simulink library "inp"  (R2021b)
settings: Solver=VariableStepAuto  StartTime=0.0  StopTime=10.0  RelTol=1e-3
undefined symbols (not defined in the file): C_TASK_5MS_S, FALSE, KINP_AcoreReadyToSlp_flg_ovrdflg, KINP_AcoreReadyToSlp_flg_ovrdval, KINP_AllowMovThd_OTA_enum_ovrdflg, KINP_AllowMovThd_OTA_enum_ovrdval, KINP_APSAngleTarget_Deg_ovrdflg, KINP_APSAngleTarget_Deg_ovrdval, KINP_APSDecReq_mps2_ovrdflg, KINP_APSDecReq_mps2_ovrdval, KINP_APSDecReqA_flg_ovrdflg, KINP_APSDecReqA_flg_ovrdval, KINP_APSDFLL_cm_ovrdflg, KINP_APSDFLL_cm_ovrdval, KINP_APSDFLR_cm_ovrdflg, KINP_APSDFLR_cm_ovrdval, KINP_APSDRLL_cm_ovrdflg, KINP_APSDRLL_cm_ovrdval, KINP_APSDRLR_cm_ovrdflg, KINP_APSDRLR_cm_ovrdval, KINP_APSExitCondition_enum_ovrdflg, KINP_APSExitCondition_enum_ovrdval, KINP_APSHWVer_enum_ovrdflg, KINP_APSHWVer_enum_ovrdval, KINP_APSProgressPCT_pct_ovrdflg, KINP_APSProgressPCT_pct_ovrdval, KINP_APSPwrReq_enum_ovrdflg, KINP_APSPwrReq_enum_ovrdval, KINP_APSReq_enum_ovrdflg, KINP_APSReq_enum_ovrdval, KINP_APSRQDisplay_enum_ovrdflg, KINP_APSRQDisplay_enum_ovrdval, KINP_APSRqEPASCtrl_flg_ovrdflg, KINP_APSRqEPASCtrl_flg_ovrdval, KINP_APSShiftPosnReq_enum_ovrdval, KINP_APSShiftPosnReq_enum_ovrflg, KINP_APSSpeedCMD_kph_ovrdval, KINP_APSSpeedCMD_kph_ovrflg, KINP_APSStaSystem_enum_ovrdflg, KINP_APSStaSystem_enum_ovrdval, KINP_APSSWVer_enum_ovrdflg, KINP_APSSWVer_enum_ovrdval, KINP_APSVMCReqA_flg_ovrdval, KINP_APSVMCReqA_flg_ovrflg, KINP_APSVRqEPASCtrl_flg_ovrdflg, KINP_APSVRqEPASCtrl_flg_ovrdval, KINP_AuxBattVolmV_mV_ovrdflg, KINP_AuxBattVolmV_mV_ovrdval, KINP_CAASSta_enum_ovrdflg, KINP_CAASSta_enum_ovrdval, KINP_CAASVMCReqA_flg_ovrdval, KINP_CAASVMCReqA_flg_ovrflg, KINP_CAN1BusOff_flg_ovrdflg, KINP_CAN1BusOff_flg_ovrdval, KINP_CAN2BusOff_flg_ovrdflg, KINP_CAN2BusOff_flg_ovrdval, KINP_CAN3BusOff_flg_ovrdflg, KINP_CAN3BusOff_flg_ovrdval, KINP_CAN4BusOff_flg_ovrdflg, KINP_CAN4BusOff_flg_ovrdval ... (+152)
libraries: FVT_lib x1037, hcu_lib x1
(part 1 of 34)
settings Model: Creator=13168  LastModifiedBy=FVT23118
settings SolverCC: AlgebraicLoopSolver=TrustRegion
settings DataIOCC: SaveFormat=Array  SignalLoggingSaveFormat=ModelDataLogs  ReturnWorkspaceOutputs=off
settings OptimizationCC: BlockReduction=off  BooleanDataType=off
settings DebuggingCC: SaveWithParameterizedLinksMsg=none  UnderspecifiedInitializationDetection=Classic  MergeDetectMultiDrivingBlocksExec=none  SignalResolutionControl=TryResolveAllWithWarning  SFMachineParentedDataDiag=warning
settings HardwareCC: TargetUnknown=on
settings ModelReferenceCC: PropagateSignalLabelsOutOfModel=off
settings SFSimCC: SimUseLocalCustomCode=off
settings ConfigComp: CovMetricSettings=dw  CovSaveCumulativeToWorkspaceVar=on  CovSaveSingleToWorkspaceVar=on

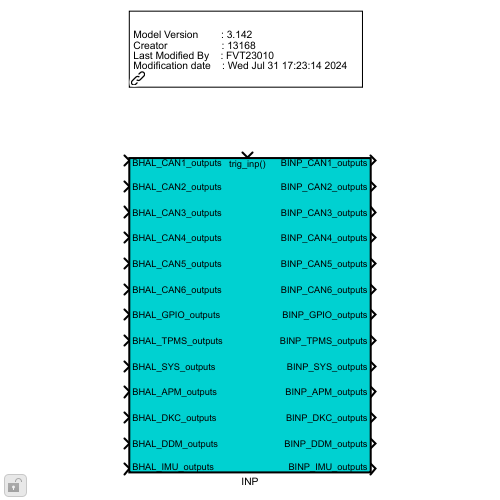
[thumbnail: Simulink's stored preview of the top-level diagram]
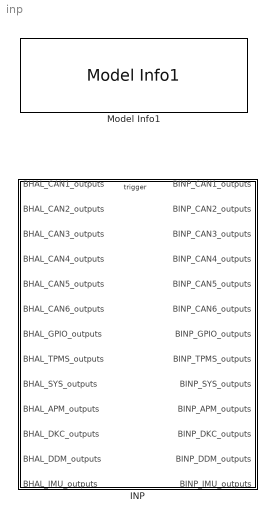
== system inp ==
  INP : Subsystem  TreatAsAtomicUnit=on
      settings: RTWSystemCode=Nonreusable function  RTWFcnNameOpts=Use subsystem name  RTWFileNameOpts=Use subsystem name
  Model Info1 : hcu_lib/Model Info1  BlockCM=None  Frame=on  DisplayStringWithTags=|  HorizontalTextAlignment=Left  LeftAlignmentValue=0.02  SourceBlockDiagram=hcu_lib  TagMaxNumber=20
      | Model Version        : %<ModelVersion>
      | Creator                   : %<Creator>
      | Last Modified By    : %<LastModifiedBy>
      | Modification date    : %<LastModificationDate>
      settings: SourceProductName=HCU Relative Block Library

== system inp/INP ==
  BHAL_CAN1_outputs : Inport  OutDataTypeStr=Bus: BHAL_CAN1_outputs
  BHAL_CAN2_outputs : Inport  Port=2  OutDataTypeStr=Bus: BHAL_CAN2_outputs
  BHAL_CAN3_outputs : Inport  Port=3  OutDataTypeStr=Bus: BHAL_CAN3_outputs
  BHAL_CAN4_outputs : Inport  Port=4  OutDataTypeStr=Bus: BHAL_CAN4_outputs
  BHAL_CAN5_outputs : Inport  Port=5  OutDataTypeStr=Bus: BHAL_CAN5_outputs
  BHAL_CAN6_outputs : Inport  Port=6  OutDataTypeStr=Bus: BHAL_CAN6_outputs
  BHAL_GPIO_outputs : Inport  Port=7  OutDataTypeStr=Bus: BHAL_GPIO_outputs
  BHAL_TPMS_outputs : Inport  Port=8  OutDataTypeStr=Bus: BHAL_TPMS_outputs
  BHAL_SYS_outputs : Inport  Port=9  OutDataTypeStr=Bus: BHAL_SYS_outputs
  BHAL_APM_outputs : Inport  Port=10  OutDataTypeStr=Bus: BHAL_APM_outputs
  BHAL_DKC_outputs : Inport  Port=11  OutDataTypeStr=Bus: BHAL_DKC_outputs
  BHAL_DDM_outputs : Inport  Port=12  OutDataTypeStr=Bus: BHAL_DDM_outputs
  BHAL_IMU_outputs : Inport  Port=13  OutDataTypeStr=Bus: BHAL_IMU_outputs
  trig_inp : TriggerPort  TriggerType=function-call  VariantControl=(inherit)
  APM : Subsystem
  CAN1 : Subsystem
  CAN2 : Subsystem
  CAN3 : Subsystem
  CAN4 : Subsystem
  CAN5 : Subsystem
  CAN6 : Subsystem
  DDM : Subsystem
  DKC : Subsystem
  GPIO : Subsystem
  IMU : Subsystem
  SYS : Subsystem
  TPMS : Subsystem
  BINP_CAN1_outputs : Outport  OutDataTypeStr=Bus: BINP_CAN1_outputs
  BINP_CAN2_outputs : Outport  Port=2  OutDataTypeStr=Bus: BINP_CAN2_outputs
  BINP_CAN3_outputs : Outport  Port=3  OutDataTypeStr=Bus: BINP_CAN3_outputs
  BINP_CAN4_outputs : Outport  Port=4  OutDataTypeStr=Bus: BINP_CAN4_outputs
  BINP_CAN5_outputs : Outport  Port=5  OutDataTypeStr=Bus: BINP_CAN5_outputs
  BINP_CAN6_outputs : Outport  Port=6  OutDataTypeStr=Bus: BINP_CAN6_outputs
  BINP_GPIO_outputs : Outport  Port=7  OutDataTypeStr=Bus: BINP_GPIO_outputs
  BINP_TPMS_outputs : Outport  Port=8  OutDataTypeStr=Bus: BINP_TPMS_outputs
  BINP_SYS_outputs : Outport  Port=9  OutDataTypeStr=Bus: BINP_SYS_outputs
  BINP_APM_outputs : Outport  Port=10  OutDataTypeStr=Bus: BINP_APM_outputs
  BINP_DKC_outputs : Outport  Port=11  OutDataTypeStr=Bus: BINP_DKC_outputs
  BINP_DDM_outputs : Outport  Port=12  OutDataTypeStr=Bus: BINP_DDM_outputs
  BINP_IMU_outputs : Outport  Port=13  OutDataTypeStr=Bus: BINP_IMU_outputs
  wires:
  BHAL_CAN1_outputs/1 -> CAN1/1(BHAL_CAN1_outputs)
  CAN1/1(INP_CAN1_outputs) -> BINP_CAN1_outputs/1
  BHAL_CAN2_outputs/1 -> CAN2/1(BHAL_CAN2_outputs)
  CAN2/1(INP_CAN2_outputs) -> BINP_CAN2_outputs/1
  BHAL_CAN3_outputs/1 -> CAN3/1(BHAL_CAN3_outputs)
  CAN3/1(INP_CAN3_outputs) -> BINP_CAN3_outputs/1
  BHAL_CAN4_outputs/1 -> CAN4/1(BHAL_CAN4_outputs)
  CAN4/1(INP_CAN4_outputs) -> BINP_CAN4_outputs/1
  GPIO/1(INP_GPIO_outputs) -> BINP_GPIO_outputs/1
  CAN5/1(INP_CAN5_outputs) -> BINP_CAN5_outputs/1
  BHAL_CAN5_outputs/1 -> CAN5/1(BHAL_CAN5_outputs)
  BHAL_GPIO_outputs/1 -> GPIO/1(BHAL_GPIO_outputs)
  BHAL_TPMS_outputs/1 -> TPMS/1(BHAL_TPMS_outputs)
  TPMS/1(BINP_TPMS_outputs) -> BINP_TPMS_outputs/1
  SYS/1(BINP_SYS_outputs) -> BINP_SYS_outputs/1
  BHAL_SYS_outputs/1 -> SYS/1(BHAL_SYS_outputs)
  BHAL_APM_outputs/1 -> APM/1(BHAL_APM_outputs)
  APM/1(BINP_APM_outputs) -> BINP_APM_outputs/1
  BHAL_DKC_outputs/1 -> DKC/1(BHAL_DKC_outputs)
  DKC/1(BINP_DKC_outputs) -> BINP_DKC_outputs/1
  BHAL_DDM_outputs/1 -> DDM/1(BHAL_DDM_outputs)
  DDM/1(BINP_DDM_outputs) -> BINP_DDM_outputs/1
  BHAL_IMU_outputs/1 -> IMU/1(BHAL_IMU_outputs)
  IMU/1(BINP_IMU_outputs) -> BINP_IMU_outputs/1
  BHAL_CAN6_outputs/1 -> CAN6/1(BHAL_CAN6_outputs)
  CAN6/1(INP_CAN6_outputs) -> BINP_CAN6_outputs/1

== system inp/INP/APM ==
  BHAL_APM_outputs : Inport  OutDataTypeStr=Bus: BHAL_APM_outputs
  Bus Creator : BusCreator  Inputs=58
  Bus Selector : BusSelector  OutputSignals=VHAL_PASDRMR_cm,VHAL_PASDRML_cm,VHAL_PASDRCR_cm,VHAL_PASDRCL_cm,VHAL_PASDFMR_cm,VHAL_PASDFML_cm,VHAL_PASDFCR_cm,VHAL_PASDFCL_cm,VHAL_APSDRLR_cm,VHAL_APSDRLL_cm,VHAL_APSDFLR_cm,VHAL_APSDFLL_cm,VHAL_PASAFCL_enum,VHAL_PASARMR_enum,VHAL_PASARML_enum,VHAL_PASARCR_enum,VHAL_PASARCL_enum,VHAL_PASAFMR_enum,VHAL_PASAFML_enum,VHAL_PASAFCR_enum,VHAL_USSStaRMR_flg,VHAL_USSStaRML_flg,VHAL_USSStaRLR_flg,VHAL_USSStaRLL_flg,VHAL_USSStaRCR_flg,VHAL_USSStaRCL_flg,VHAL_USSStaFMR_flg,VHAL_USSStaFML_flg,VHAL_USSStaFLR_flg,VHAL_USSStaFLL_flg,VHAL_USSStaFCR_flg,VHAL_USSStaFCL_flg,VHAL_Chime_enum,VHAL_SNSRLayout_enum,VHAL_StaFSya_flg,VHAL_ModOperation_enum,VHAL_APSProgressPCT_pct,VHAL_APSRQDisplay_enum,VHAL_APSSWVer_enum,VHAL_APSHWVer_enum,VHAL_APSExitCondition_enum,VHAL_APSAngleTarget_Deg,VHAL_APSStaSystem_enum,VHAL_APSVRqEPASCtrl_flg,VHAL_APSRqEPASCtrl_flg,VHAL_APSReq_enum,VHAL_APSDecReq_mps2,VHAL_APSDecReqA_flg,VHAL_APSShiftPosnReq_enum,VHAL_APSSpeedCMD_kph,VHAL_APSVMCReqA_flg,VHAL_CAASSta_enum,VHAL_CAASVMCReqA_flg,VHAL_APSPwrReq_enum,VHAL_RAPSBCMLockReq_flg,VHAL_RAPSBCMLamp_enum,VHAL_RAPSErrWarnSta_enum,VHAL_RAPSErrLv1_flg
  Data Type Conversion{,16,18..19,21..24,28..33,37,47..48,51,54,57} (20 alike) : DataTypeConversion  OutDataTypeStr=boolean
  Data Type Conversion{1..7,12..15,17,20,25..27,34..36,38,41..44,46,49,52..53,55..56} (30 alike) : DataTypeConversion  OutDataTypeStr=uint8
  Data Type Conversion{8..11} (4 alike) : DataTypeConversion  OutDataTypeStr=uint16
  Data Type Conversion{39..40,45,50} (4 alike) : DataTypeConversion  OutDataTypeStr=single
  Subsystem : Subsystem
  Subsystem1 : Subsystem
  Subsystem10 : Subsystem
  Subsystem11 : Subsystem
  Subsystem12 : Subsystem
  Subsystem13 : Subsystem
  Subsystem14 : Subsystem
  Subsystem15 : Subsystem
  Subsystem16 : Subsystem
  Subsystem17 : Subsystem
  Subsystem18 : Subsystem
  Subsystem19 : Subsystem
  Subsystem2 : Subsystem
  Subsystem20 : Subsystem
  Subsystem21 : Subsystem
  Subsystem22 : Subsystem
  Subsystem23 : Subsystem
  Subsystem24 : Subsystem
  Subsystem25 : Subsystem
  Subsystem26 : Subsystem
  Subsystem27 : Subsystem
  Subsystem28 : Subsystem
  Subsystem29 : Subsystem
  Subsystem3 : Subsystem
  Subsystem30 : Subsystem
  Subsystem31 : Subsystem
  Subsystem32 : Subsystem
  Subsystem33 : Subsystem
  Subsystem34 : Subsystem
  Subsystem35 : Subsystem
  Subsystem36 : Subsystem
  Subsystem37 : Subsystem
  Subsystem38 : Subsystem
  Subsystem39 : Subsystem
  Subsystem4 : Subsystem
  Subsystem40 : Subsystem
  Subsystem41 : Subsystem
  Subsystem42 : Subsystem
  Subsystem43 : Subsystem
  Subsystem44 : Subsystem
  Subsystem45 : Subsystem
  Subsystem46 : Subsystem
  Subsystem47 : Subsystem
  Subsystem48 : Subsystem
  Subsystem49 : Subsystem
  Subsystem5 : Subsystem
  Subsystem50 : Subsystem
  Subsystem51 : Subsystem
  Subsystem52 : Subsystem
  Subsystem53 : Subsystem
  Subsystem54 : Subsystem
  Subsystem55 : Subsystem
  Subsystem56 : Subsystem
  Subsystem57 : Subsystem
  Subsystem6 : Subsystem
  Subsystem7 : Subsystem
  Subsystem8 : Subsystem
  Subsystem9 : Subsystem
  BINP_APM_outputs : Outport  OutDataTypeStr=Bus: BINP_APM_outputs
  wires:
  BHAL_APM_outputs/1 -> Bus Selector/1
  Data Type Conversion13/1 -> Bus Creator/16  "VINP_PASARCR_enum"
  Data Type Conversion36/1 -> Bus Creator/33  "VINP_Chime_enum"
  Data Type Conversion20/1 -> Bus Creator/1  "VINP_PASDRMR_cm"
  Data Type Conversion1/1 -> Bus Creator/2  "VINP_PASDRML_cm"
  Data Type Conversion12/1 -> Bus Creator/14  "VINP_PASARMR_enum"
  Data Type Conversion9/1 -> Bus Creator/11  "VINP_APSDFLR_cm"
  Data Type Conversion15/1 -> Bus Creator/15  "VINP_PASARML_enum"
  Bus Creator/1 -> BINP_APM_outputs/1
  Data Type Conversion30/1 -> Bus Creator/24  "VINP_USSStaRLL_flg"
  Data Type Conversion25/1 -> Bus Creator/20  "VINP_PASAFCR_enum"
  Data Type Conversion2/1 -> Bus Creator/4  "VINP_PASDRCL_cm"
  Data Type Conversion18/1 -> Bus Creator/22  "VINP_USSStaRML_flg"
  Data Type Conversion14/1 -> Bus Creator/13  "VINP_PASAFCL_enum"
  Data Type Conversion7/1 -> Bus Creator/7  "VINP_PASDFCR_cm"
  Data Type Conversion17/1 -> Bus Creator/18  "VINP_PASAFMR_enum"
  Data Type Conversion34/1 -> Bus Creator/34  "VINP_SNSRLayout_enum"
  Data Type Conversion35/1 -> Bus Creator/36  "VINP_ModOperation_enum"
  Data Type Conversion/1 -> Bus Creator/21  "VINP_USSStaRMR_flg"
  Data Type Conversion6/1 -> Bus Creator/5  "VINP_PASDFMR_cm"
  Data Type Conversion32/1 -> Bus Creator/30  "VINP_USSStaFLL_flg"
  Data Type Conversion4/1 -> Bus Creator/6  "VINP_PASDFML_cm"
  Data Type Conversion10/1 -> Bus Creator/9  "VINP_APSDRLR_cm"
  Data Type Conversion8/1 -> Bus Creator/10  "VINP_APSDRLL_cm"
  Data Type Conversion5/1 -> Bus Creator/8  "VINP_PASDFCL_cm"
  Data Type Conversion33/1 -> Bus Creator/35  "VINP_StaFSya_flg"
  Data Type Conversion11/1 -> Bus Creator/12  "VINP_APSDFLL_cm"
  Data Type Conversion31/1 -> Bus Creator/29  "VINP_USSStaFLR_flg"
  Data Type Conversion3/1 -> Bus Creator/3  "VINP_PASDRCR_cm"
  Data Type Conversion28/1 -> Bus Creator/32  "VINP_USSStaFCL_flg"
  Data Type Conversion21/1 -> Bus Creator/26  "VINP_USSStaRCL_flg"
  Data Type Conversion22/1 -> Bus Creator/27  "VINP_USSStaFMR_flg"
  Data Type Conversion27/1 -> Bus Creator/19  "VINP_PASAFML_enum"
  Data Type Conversion19/1 -> Bus Creator/25  "VINP_USSStaRCR_flg"
  Data Type Conversion26/1 -> Bus Creator/17  "VINP_PASARCL_enum"
  Data Type Conversion23/1 -> Bus Creator/28  "VINP_USSStaFML_flg"
  Data Type Conversion29/1 -> Bus Creator/23  "VINP_USSStaRLR_flg"
  Data Type Conversion24/1 -> Bus Creator/31  "VINP_USSStaFCR_flg"
  Subsystem/1(Out1) -> Data Type Conversion20/1
  Bus Selector/1 -> Subsystem/1(In1)  "<VHAL_PASDRMR_cm>"
  Subsystem1/1(Out1) -> Data Type Conversion1/1
  Bus Selector/2 -> Subsystem1/1(In1)  "<VHAL_PASDRML_cm>"
  Subsystem2/1(Out1) -> Data Type Conversion3/1
  Bus Selector/3 -> Subsystem2/1(In1)  "<VHAL_PASDRCR_cm>"
  Subsystem3/1(Out1) -> Data Type Conversion2/1
  Bus Selector/4 -> Subsystem3/1(In1)  "<VHAL_PASDRCL_cm>"
  Subsystem4/1(Out1) -> Data Type Conversion6/1
  Bus Selector/5 -> Subsystem4/1(In1)  "<VHAL_PASDFMR_cm>"
  Subsystem5/1(Out1) -> Data Type Conversion4/1
  Bus Selector/6 -> Subsystem5/1(In1)  "<VHAL_PASDFML_cm>"
  Subsystem6/1(Out1) -> Data Type Conversion7/1
  Bus Selector/7 -> Subsystem6/1(In1)  "<VHAL_PASDFCR_cm>"
  Bus Selector/8 -> Subsystem7/1(In1)  "<VHAL_PASDFCL_cm>"
  Subsystem7/1(Out1) -> Data Type Conversion5/1
  Bus Selector/9 -> Subsystem8/1(In1)  "<VHAL_APSDRLR_cm>"
  Subsystem8/1(Out1) -> Data Type Conversion10/1
  Bus Selector/10 -> Subsystem9/1(In1)  "<VHAL_APSDRLL_cm>"
  Subsystem9/1(Out1) -> Data Type Conversion8/1
  Bus Selector/11 -> Subsystem10/1(In1)  "<VHAL_APSDFLR_cm>"
  Subsystem10/1(Out1) -> Data Type Conversion9/1
  Subsystem11/1(Out1) -> Data Type Conversion11/1
  Bus Selector/12 -> Subsystem11/1(In1)  "<VHAL_APSDFLL_cm>"
  Bus Selector/13 -> Subsystem12/1(In1)  "<VHAL_PASAFCL_enum>"
  Subsystem12/1(Out1) -> Data Type Conversion14/1
  Subsystem13/1(Out1) -> Data Type Conversion12/1
  Bus Selector/14 -> Subsystem13/1(In1)  "<VHAL_PASARMR_enum>"
  Subsystem14/1(Out1) -> Data Type Conversion15/1
  Bus Selector/15 -> Subsystem14/1(In1)  "<VHAL_PASARML_enum>"
  Subsystem15/1(Out1) -> Data Type Conversion13/1
  Bus Selector/16 -> Subsystem15/1(In1)  "<VHAL_PASARCR_enum>"
  Subsystem16/1(Out1) -> Data Type Conversion26/1
  Bus Selector/17 -> Subsystem16/1(In1)  "<VHAL_PASARCL_enum>"
  Bus Selector/18 -> Subsystem17/1(In1)  "<VHAL_PASAFMR_enum>"
  Subsystem17/1(Out1) -> Data Type Conversion17/1
  Subsystem18/1(Out1) -> Data Type Conversion27/1
  Bus Selector/19 -> Subsystem18/1(In1)  "<VHAL_PASAFML_enum>"
  Bus Selector/20 -> Subsystem19/1(In1)  "<VHAL_PASAFCR_enum>"
  Subsystem19/1(Out1) -> Data Type Conversion25/1
  Bus Selector/21 -> Subsystem20/1(In1)  "<VHAL_USSStaRMR_flg>"
  Subsystem20/1(Out1) -> Data Type Conversion/1
  Bus Selector/22 -> Subsystem21/1(In1)  "<VHAL_USSStaRML_flg>"
  Subsystem21/1(Out1) -> Data Type Conversion18/1
  Bus Selector/23 -> Subsystem22/1(In1)  "<VHAL_USSStaRLR_flg>"
  Subsystem22/1(Out1) -> Data Type Conversion29/1
  Bus Selector/24 -> Subsystem23/1(In1)  "<VHAL_USSStaRLL_flg>"
  Subsystem23/1(Out1) -> Data Type Conversion30/1
  Bus Selector/25 -> Subsystem24/1(In1)  "<VHAL_USSStaRCR_flg>"
  Subsystem24/1(Out1) -> Data Type Conversion19/1
  Bus Selector/26 -> Subsystem25/1(In1)  "<VHAL_USSStaRCL_flg>"
  Subsystem25/1(Out1) -> Data Type Conversion21/1
  Bus Selector/27 -> Subsystem26/1(In1)  "<VHAL_USSStaFMR_flg>"
  Subsystem26/1(Out1) -> Data Type Conversion22/1
  Bus Selector/28 -> Subsystem27/1(In1)  "<VHAL_USSStaFML_flg>"
  Subsystem27/1(Out1) -> Data Type Conversion23/1
  Bus Selector/29 -> Subsystem28/1(In1)  "<VHAL_USSStaFLR_flg>"
  Subsystem28/1(Out1) -> Data Type Conversion31/1
  Bus Selector/30 -> Subsystem29/1(In1)  "<VHAL_USSStaFLL_flg>"
  Subsystem29/1(Out1) -> Data Type Conversion32/1
  Bus Selector/31 -> Subsystem30/1(In1)  "<VHAL_USSStaFCR_flg>"
  Subsystem30/1(Out1) -> Data Type Conversion24/1
  Bus Selector/32 -> Subsystem31/1(In1)  "<VHAL_USSStaFCL_flg>"
  Subsystem31/1(Out1) -> Data Type Conversion28/1
  Bus Selector/33 -> Subsystem32/1(In1)  "<VHAL_Chime_enum>"
  Subsystem32/1(Out1) -> Data Type Conversion36/1
  Bus Selector/34 -> Subsystem33/1(In1)  "<VHAL_SNSRLayout_enum>"
  Subsystem33/1(Out1) -> Data Type Conversion34/1
  Bus Selector/35 -> Subsystem34/1(In1)  "<VHAL_StaFSya_flg>"
  Subsystem34/1(Out1) -> Data Type Conversion33/1
  Subsystem35/1(Out1) -> Data Type Conversion35/1
  Bus Selector/36 -> Subsystem35/1(In1)  "<VHAL_ModOperation_enum>"
  Subsystem40/1(Out1) -> Data Type Conversion40/1
  Data Type Conversion40/1 -> Bus Creator/37  "VINP_APSProgressPCT_pct"
  Subsystem41/1(Out1) -> Data Type Conversion41/1
  Data Type Conversion41/1 -> Bus Creator/38  "VINP_APSRQDisplay_enum"
  Data Type Conversion42/1 -> Bus Creator/39  "VINP_APSSWVer_enum"
  Subsystem42/1(Out1) -> Data Type Conversion42/1
  Subsystem43/1(Out1) -> Data Type Conversion43/1
  Data Type Conversion43/1 -> Bus Creator/40  "VINP_APSHWVer_enum"
  Data Type Conversion44/1 -> Bus Creator/41  "VINP_APSExitCondition_enum"
  Subsystem44/1(Out1) -> Data Type Conversion44/1
  Data Type Conversion45/1 -> Bus Creator/42  "VINP_APSAngleTarget_Deg"
  Subsystem45/1(Out1) -> Data Type Conversion45/1
  Subsystem46/1(Out1) -> Data Type Conversion46/1
  Data Type Conversion46/1 -> Bus Creator/43  "VINP_APSStaSystem_enum"
  Subsystem47/1(Out1) -> Data Type Conversion47/1
  Data Type Conversion47/1 -> Bus Creator/44  "VINP_APSVRqEPASCtrl_flg"
  Data Type Conversion48/1 -> Bus Creator/45  "VINP_APSRqEPASCtrl_flg"
  Subsystem48/1(Out1) -> Data Type Conversion48/1
  Data Type Conversion49/1 -> Bus Creator/46  "VINP_APSReq_enum"
  Subsystem49/1(Out1) -> Data Type Conversion49/1
  Subsystem50/1(Out1) -> Data Type Conversion50/1
  Data Type Conversion50/1 -> Bus Creator/47  "VINP_APSDecReq_mps2"
  Subsystem51/1(Out1) -> Data Type Conversion51/1
  Data Type Conversion51/1 -> Bus Creator/48  "VINP_APSDecReqA_flg"
  Subsystem52/1(Out1) -> Data Type Conversion52/1
  Subsystem36/1(Out1) -> Data Type Conversion37/1
  Data Type Conversion39/1 -> Bus Creator/50  "VINP_APSSpeedCMD_kph"
  Data Type Conversion37/1 -> Bus Creator/51  "VINP_APSVMCReqA_flg"
  Subsystem38/1(Out1) -> Data Type Conversion39/1
  Subsystem37/1(Out1) -> Data Type Conversion38/1
  Data Type Conversion38/1 -> Bus Creator/49  "VINP_APSShiftPosnReq_enum"
  Data Type Conversion52/1 -> Bus Creator/52  "VINP_CAASSta_enum"
  Bus Selector/37 -> Subsystem40/1(In1)  "<VHAL_APSProgressPCT_pct>"
  Bus Selector/38 -> Subsystem41/1(In1)  "<VHAL_APSRQDisplay_enum>"
  Bus Selector/39 -> Subsystem42/1(In1)  "<VHAL_APSSWVer_enum>"
  Bus Selector/40 -> Subsystem43/1(In1)  "<VHAL_APSHWVer_enum>"
  Bus Selector/41 -> Subsystem44/1(In1)  "<VHAL_APSExitCondition_enum>"
  Bus Selector/42 -> Subsystem45/1(In1)  "<VHAL_APSAngleTarget_Deg>"
  Bus Selector/43 -> Subsystem46/1(In1)  "<VHAL_APSStaSystem_enum>"
  Bus Selector/44 -> Subsystem47/1(In1)  "<VHAL_APSVRqEPASCtrl_flg>"
  Bus Selector/45 -> Subsystem48/1(In1)  "<VHAL_APSRqEPASCtrl_flg>"
  Bus Selector/46 -> Subsystem49/1(In1)  "<VHAL_APSReq_enum>"
  Bus Selector/47 -> Subsystem50/1(In1)  "<VHAL_APSDecReq_mps2>"
  Bus Selector/48 -> Subsystem51/1(In1)  "<VHAL_APSDecReqA_flg>"
  Bus Selector/49 -> Subsystem37/1(In1)  "<VHAL_APSShiftPosnReq_enum>"
  Bus Selector/50 -> Subsystem38/1(In1)  "<VHAL_APSSpeedCMD_kph>"
  Bus Selector/51 -> Subsystem36/1(In1)  "<VHAL_APSVMCReqA_flg>"
  Bus Selector/52 -> Subsystem52/1(In1)  "<VHAL_CAASSta_enum>"
  Subsystem39/1(Out1) -> Data Type Conversion16/1
  Bus Selector/53 -> Subsystem39/1(In1)  "<VHAL_CAASVMCReqA_flg>"
  Data Type Conversion16/1 -> Bus Creator/53  "VINP_CAASVMCReqA_flg"
  Subsystem53/1(Out1) -> Data Type Conversion53/1
  Subsystem55/1(Out1) -> Data Type Conversion54/1
  Subsystem54/1(Out1) -> Data Type Conversion55/1
  Bus Selector/54 -> Subsystem53/1(In1)  "<VHAL_APSPwrReq_enum>"
  Bus Selector/55 -> Subsystem55/1(In1)  "<VHAL_RAPSBCMLockReq_flg>"
  Bus Selector/56 -> Subsystem54/1(In1)  "<VHAL_RAPSBCMLamp_enum>"
  Data Type Conversion53/1 -> Bus Creator/54  "VINP_APSPwrReq_enum"
  Data Type Conversion54/1 -> Bus Creator/55  "VINP_RAPSBCMLockReq_flg"
  Data Type Conversion55/1 -> Bus Creator/56  "VINP_RAPSBCMLamp_enum"
  Data Type Conversion56/1 -> Bus Creator/57  "VINP_RAPSErrWarnSta_enum"
  Data Type Conversion57/1 -> Bus Creator/58  "VINP_RAPSErrLv1_flg"
  Bus Selector/57 -> Subsystem57/1(In1)  "<VHAL_RAPSErrWarnSta_enum>"
  Bus Selector/58 -> Subsystem56/1(In1)  "<VHAL_RAPSErrLv1_flg>"
  Subsystem57/1(Out1) -> Data Type Conversion56/1
  Subsystem56/1(Out1) -> Data Type Conversion57/1

== system inp/INP/CAN1 ==
  BHAL_CAN1_outputs : Inport
  CommunicationCheck : Subsystem
  CreateBus : Subsystem
  SignalCheck : Subsystem
  ctasktime : Constant  Value=C_TASK_5MS_S  OutDataTypeStr=single
  INP_CAN1_outputs : Outport
  wires:
  CreateBus/1(BINP_outputs) -> INP_CAN1_outputs/1
  CommunicationCheck/1(inp_CanValid_bus) -> [inp_CanValid_bus], SignalCheck/1(inp_CanValid_bus)
  [inp_CanValid_bus] -> CreateBus/1(inp_CanValid_bus)
  BHAL_CAN1_outputs/1 -> CommunicationCheck/1(BHAL_outputs), SignalCheck/3(BHAL_outputs)
  SignalCheck/1(inp_Hal_bus) -> CreateBus/2(inp_Hal_bus)
  ctasktime/1 -> SignalCheck/2(TASK_TIME_S)

== system inp/INP/CAN2 ==
  BHAL_CAN2_outputs : Inport
  CommunicationCheck : Subsystem
  CreateBus : Subsystem
  SignalCheck : Subsystem
  ctasktime : Constant  Value=C_TASK_5MS_S  OutDataTypeStr=single
  INP_CAN2_outputs : Outport
  wires:
  CreateBus/1(BINP_outputs) -> INP_CAN2_outputs/1
  CommunicationCheck/1(inp_CanValid_bus) -> [inp_CanValid_bus], SignalCheck/1(inp_CanValid_bus)
  [inp_CanValid_bus] -> CreateBus/1(inp_CanValid_bus)
  BHAL_CAN2_outputs/1 -> CommunicationCheck/1(BHAL_outputs), SignalCheck/3(BHAL_outputs)
  SignalCheck/1(inp_Hal_bus) -> CreateBus/2(inp_Hal_bus)
  ctasktime/1 -> SignalCheck/2(TASK_TIME_S)

== system inp/INP/CAN3 ==
  BHAL_CAN3_outputs : Inport
  CommunicationCheck : Subsystem
  CreateBus : Subsystem
  SignalCheck : Subsystem
  ctasktime : Constant  Value=C_TASK_5MS_S  OutDataTypeStr=single
  INP_CAN3_outputs : Outport
  wires:
  CreateBus/1(BINP_outputs) -> INP_CAN3_outputs/1
  CommunicationCheck/1(inp_CanValid_bus) -> [inp_CanValid_bus], SignalCheck/1(inp_CanValid_bus)
  [inp_CanValid_bus] -> CreateBus/1(inp_CanValid_bus)
  BHAL_CAN3_outputs/1 -> CommunicationCheck/1(BHAL_outputs), SignalCheck/3(BHAL_outputs)
  SignalCheck/1(inp_Hal_bus) -> CreateBus/2(inp_Hal_bus)
  ctasktime/1 -> SignalCheck/2(TASK_TIME_S)

== system inp/INP/CAN4 ==
  BHAL_CAN4_outputs : Inport
  CommunicationCheck : Subsystem
  CreateBus : Subsystem
  SignalCheck : Subsystem
  ctasktime : Constant  Value=C_TASK_5MS_S  OutDataTypeStr=single
  INP_CAN4_outputs : Outport
  wires:
  CreateBus/1(BINP_outputs) -> INP_CAN4_outputs/1
  CommunicationCheck/1(inp_CanValid_bus) -> [inp_CanValid_bus], SignalCheck/1(inp_CanValid_bus)
  [inp_CanValid_bus] -> CreateBus/1(inp_CanValid_bus)
  BHAL_CAN4_outputs/1 -> CommunicationCheck/1(BHAL_outputs), SignalCheck/3(BHAL_outputs)
  SignalCheck/1(inp_Hal_bus) -> CreateBus/2(inp_Hal_bus)
  ctasktime/1 -> SignalCheck/2(TASK_TIME_S)

== system inp/INP/CAN5 ==
  BHAL_CAN5_outputs : Inport
  CommunicationCheck : Subsystem
  CreateBus : Subsystem
  SignalCheck : Subsystem
  ctasktime : Constant  Value=C_TASK_5MS_S  OutDataTypeStr=single
  INP_CAN5_outputs : Outport
  wires:
  CreateBus/1(BINP_outputs) -> INP_CAN5_outputs/1
  CommunicationCheck/1(inp_CanValid_bus) -> [inp_CanValid_bus], SignalCheck/1(inp_CanValid_bus)
  [inp_CanValid_bus] -> CreateBus/1(inp_CanValid_bus)
  BHAL_CAN5_outputs/1 -> CommunicationCheck/1(BHAL_outputs), SignalCheck/3(BHAL_outputs)
  SignalCheck/1(inp_Hal_bus) -> CreateBus/2(inp_Hal_bus)
  ctasktime/1 -> SignalCheck/2(TASK_TIME_S)

== system inp/INP/CAN6 ==
  BHAL_CAN6_outputs : Inport
  CommunicationCheck : Subsystem
  CreateBus : Subsystem
  SignalCheck : Subsystem
  ctasktime : Constant  Value=C_TASK_5MS_S  OutDataTypeStr=single
  INP_CAN6_outputs : Outport
  wires:
  CreateBus/1(BINP_outputs) -> INP_CAN6_outputs/1
  CommunicationCheck/1(inp_CanValid_bus) -> [inp_CanValid_bus], SignalCheck/1(inp_CanValid_bus)
  [inp_CanValid_bus] -> CreateBus/1(inp_CanValid_bus)
  BHAL_CAN6_outputs/1 -> CommunicationCheck/1(BHAL_outputs), SignalCheck/3(BHAL_outputs)
  SignalCheck/1(inp_Hal_bus) -> CreateBus/2(inp_Hal_bus)
  ctasktime/1 -> SignalCheck/2(TASK_TIME_S)

== system inp/INP/DDM ==
  BHAL_DDM_outputs : Inport
  Bus Creator : BusCreator  Inputs=1
  Bus Selector : BusSelector  OutputSignals=VHAL_ClearDTCcmd_flg
  Data Type Conversion12 : DataTypeConversion  OutDataTypeStr=boolean
  Subsystem13 : Subsystem
  BINP_DDM_outputs : Outport
  wires:
  Bus Selector/1 -> Subsystem13/1(In1)  "<VHAL_ClearDTCcmd_flg>"
  Subsystem13/1(Out1) -> Data Type Conversion12/1
  BHAL_DDM_outputs/1 -> Bus Selector/1
  Data Type Conversion12/1 -> Bus Creator/1  "VINP_ClearDTCcmd_flg"
  Bus Creator/1 -> BINP_DDM_outputs/1

== system inp/INP/DKC ==
  BHAL_DKC_outputs : Inport  OutDataTypeStr=Bus: BHAL_DKC_outputs
  Bus Creator : BusCreator  Inputs=18
  Bus Selector : BusSelector  OutputSignals=VHAL_DKCDecReVehData_enum,VHAL_DKCDecRemotePW_enum,VHAL_DKCDecPCommandToBCM_enum,VHAL_DKCDecPCommandToPTG_enum,VHAL_DKCDecPDKeyAreaLockUnlock_enum,VHAL_DKCDecPDKeyAreaPS_enum,VHAL_DKCDecPDKeyAreaPTG_enum,VHAL_DKCDecPDKeyWelcome_enum,VHAL_DKCDecPDkeyShowIVI_enum,VHAL_DKCDecPKeyMiss_flg,VHAL_DKCDecPKeyMode_enum,VHAL_DKCDecPUIDLowPower_flg,VHAL_TimeSNDKCFbk_cnt,VHAL_DKCDecryptionFail_flg,VHAL_NFCDoorSta_flg,VHAL_NFCLidASta_flg,VHAL_KeyFobAreaU16_enum,VHAL_UIDButtonCmd_enum
  Data Type Conversion{1..9,11} (10 alike) : DataTypeConversion  OutDataTypeStr=uint8
  Data Type Conversion10 : DataTypeConversion  OutDataTypeStr=boolean
  Data Type Conversion12 : DataTypeConversion  OutDataTypeStr=boolean
  Data Type Conversion14 : DataTypeConversion  OutDataTypeStr=boolean
  Data Type Conversion15 : DataTypeConversion  OutDataTypeStr=uint32
  Subsystem1 : Subsystem
  Subsystem10 : Subsystem
  Subsystem2 : Subsystem
  Subsystem3 : Subsystem
  BINP_DKC_outputs : Outport  OutDataTypeStr=Bus: BINP_DKC_outputs
  wires:
  Data Type Conversion15/1 -> Bus Creator/13  "VINP_TimeSNDKCFbk_cnt"
  Data Type Conversion14/1 -> Bus Creator/12  "VINP_DKCDecPUIDLowPower_flg"
  Data Type Conversion11/1 -> Bus Creator/11  "VINP_DKCDecPKeyMode_enum"
  Data Type Conversion12/1 -> Bus Creator/10  "VINP_DKCDecPKeyMiss_flg"
  Data Type Conversion9/1 -> Bus Creator/9  "VINP_DKCDecPDkeyShowIVI_enum"
  Data Type Conversion8/1 -> Bus Creator/8  "VINP_DKCDecPDKeyWelcome_enum"
  Data Type Conversion7/1 -> Bus Creator/7  "VINP_DKCDecPDKeyAreaPTG_enum"
  Data Type Conversion6/1 -> Bus Creator/6  "VINP_DKCDecPDKeyAreaPS_enum"
  Data Type Conversion5/1 -> Bus Creator/5  "VINP_DKCDecPDKeyAreaLockUnlock_enum"
  Data Type Conversion4/1 -> Bus Creator/4  "VINP_DKCDecPCommandToPTG_enum"
  Data Type Conversion3/1 -> Bus Creator/3  "VINP_DKCDecPCommandToBCM_enum"
  Data Type Conversion2/1 -> Bus Creator/2  "VINP_DKCDecRemotePW_enum"
  Data Type Conversion1/1 -> Bus Creator/1  "VINP_DKCDecReVehData_enum"
  Bus Selector/13 -> Data Type Conversion15/1  "<VHAL_TimeSNDKCFbk_cnt>"
  Bus Selector/12 -> Data Type Conversion14/1  "<VHAL_DKCDecPUIDLowPower_flg>"
  Bus Selector/11 -> Data Type Conversion11/1  "<VHAL_DKCDecPKeyMode_enum>"
  Bus Selector/10 -> Data Type Conversion12/1  "<VHAL_DKCDecPKeyMiss_flg>"
  Bus Selector/9 -> Data Type Conversion9/1  "<VHAL_DKCDecPDkeyShowIVI_enum>"
  Bus Selector/8 -> Data Type Conversion8/1  "<VHAL_DKCDecPDKeyWelcome_enum>"
  Bus Selector/7 -> Data Type Conversion7/1  "<VHAL_DKCDecPDKeyAreaPTG_enum>"
  Bus Selector/6 -> Data Type Conversion6/1  "<VHAL_DKCDecPDKeyAreaPS_enum>"
  Bus Selector/5 -> Data Type Conversion5/1  "<VHAL_DKCDecPDKeyAreaLockUnlock_enum>"
  Bus Selector/4 -> Data Type Conversion4/1  "<VHAL_DKCDecPCommandToPTG_enum>"
  Bus Selector/3 -> Data Type Conversion3/1  "<VHAL_DKCDecPCommandToBCM_enum>"
  Bus Selector/2 -> Data Type Conversion2/1  "<VHAL_DKCDecRemotePW_enum>"
  Bus Selector/1 -> Data Type Conversion1/1  "<VHAL_DKCDecReVehData_enum>"
  Bus Creator/1 -> BINP_DKC_outputs/1
  BHAL_DKC_outputs/1 -> Bus Selector/1
  Bus Selector/14 -> Data Type Conversion10/1  "<VHAL_DKCDecryptionFail_flg>"
  Data Type Conversion10/1 -> Bus Creator/14  "VINP_DKCDecryptionFail_flg"
  Bus Selector/15 -> Subsystem10/1(In1)  "<VHAL_NFCDoorSta_flg>"
  Subsystem10/1(Out1) -> Bus Creator/15  "VINP_NFCDoorSta_flg"
  Bus Selector/16 -> Subsystem1/1(In1)  "<VHAL_NFCLidASta_flg>"
  Bus Selector/17 -> Subsystem2/1(In1)  "<VHAL_KeyFobAreaU16_enum>"
  Subsystem1/1(Out1) -> Bus Creator/16  "VINP_NFCLidASta_flg"
  Subsystem2/1(Out1) -> Bus Creator/17  "VINP_KeyFobAreaU16_enum"
  Bus Selector/18 -> Subsystem3/1(In1)  "<VHAL_UIDButtonCmd_enum>"
  Subsystem3/1(Out1) -> Bus Creator/18  "VINP_UIDButtonCmd_enum"

== system inp/INP/GPIO ==
  BHAL_GPIO_outputs : Inport
  Analog : Subsystem
  Bus Selector : BusSelector  OutputSignals=VHAL_HWID1_enum,VHAL_HWID2_enum,VHAL_HWID3_enum,VHAL_HWID4_enum
  Constant : Constant  Value=C_TASK_5MS_S
  Digital : Subsystem
  UnitConverter_{1..2,5..6,10..12,69} (8 alike) : DataTypeConversion  OutDataTypeStr=uint8
  UnitConverter_{4,8..9,17..28} (15 alike) : DataTypeConversion  OutDataTypeStr=boolean
  UnitConverter_3 : DataTypeConversion  OutDataTypeStr=single
  UnitConverter_7 : DataTypeConversion  OutDataTypeStr=single
  bus_creator : BusCreator  Inputs=25
  INP_GPIO_outputs : Outport
  wires:
  Digital/9(VINP_HazardSW_flg) -> [VINP_HazardSW_flg]
  Digital/10(VINP_BrakeLampSW_flg) -> [VINP_BrakeLampSW_flg]
  Digital/8(VINP_CentralDoorLockSW_flg) -> [VINP_CentralDoorLockSW_flg]
  Analog/4(VINP_AccelPedal1VolValid_flg) -> [VINP_AccelPedal1VolValid_flg]
  Digital/11(VINP_TrunkHanSW_flg) -> [VINP_TrunkHanSW_flg]
  Digital/7(VINP_RLDoorSW_flg) -> [VINP_RLDoorSW_flg]
  Digital/6(VINP_RRDoorSW_flg) -> [VINP_RRDoorSW_flg]
  Digital/4(VINP_DrDoorSW_flg) -> [VINP_DrDoorSW_flg]
  Digital/12(VINP_SeatSW_flg) -> [VINP_SeatSW_flg]
  Analog/5(VINP_AccelPedal2VolShortHigh_enum) -> [VINP_AccelPedal2VolShortHigh_enum]
  Digital/1(VINP_BrakeSWGPIO_flg) -> [VINP_BrakeSWGPIO_flg]
  Analog/8(VINP_AccelPedal2VolValid_flg) -> [VINP_AccelPedal2VolValid_flg]
  [BHAL_outputs] -> Digital/1(BHAL_outputs)
  Analog/3(VINP_AccelPedal1Vol_V) -> [VINP_AccelPedal1Vol_V]
  Digital/5(VINP_PsDoorSW_flg) -> [VINP_PsDoorSW_flg]
  Analog/6(VINP_AccelPedal2VolShortLow_enum) -> [VINP_AccelPedal2VolShortLow_enum]
  [BHAL_outputs] -> Analog/1(BHAL_outputs)
  Digital/2(VINP_HoodSW_flg) -> [VINP_HoodSW_flg]
  Analog/1(VINP_AccelPedal1VolShortHigh_enum) -> [VINP_AccelPedal1VolShortHigh_enum]
  Analog/2(VINP_AccelPedal1VolShortLow_enum) -> [VINP_AccelPedal1VolShortLow_enum]
  Digital/3(VINP_TailgateSW_flg) -> [VINP_TailgateSW_flg]
  Analog/7(VINP_AccelPedal2Vol_V) -> [VINP_AccelPedal2Vol_V]
  Constant/1 -> Analog/2(TASK_TIME_S)
  BHAL_GPIO_outputs/1 -> [BHAL_outputs]
  [BHAL_outputs] -> Bus Selector/1
  Digital/13(VINP_CrashSignalGPIO_flg) -> [VINP_CrashSignalGPIO_flg]
  Bus Selector/1 -> [VINP_HWID1_enum]  "<VHAL_HWID1_enum>"
  Bus Selector/2 -> [VINP_HWID2_enum]  "<VHAL_HWID2_enum>"
  Bus Selector/3 -> [VINP_HWID3_enum]  "<VHAL_HWID3_enum>"
  Bus Selector/4 -> [VINP_HWID4_enum]  "<VHAL_HWID4_enum>"
  [VINP_SeatSW_flg] -> UnitConverter_28/1
  UnitConverter_10/1 -> bus_creator/23  "VINP_HWID2_enum"
  UnitConverter_12/1 -> bus_creator/25  "VINP_HWID4_enum"
  UnitConverter_23/1 -> bus_creator/15  "VINP_RLDoorSW_flg"
  [VINP_AccelPedal2VolValid_flg] -> UnitConverter_8/1
  [VINP_HWID2_enum] -> UnitConverter_10/1
  UnitConverter_28/1 -> bus_creator/20  "VINP_SeatSW_flg"
  [VINP_HWID3_enum] -> UnitConverter_11/1
  [VINP_HWID4_enum] -> UnitConverter_12/1
  UnitConverter_69/1 -> bus_creator/22  "VINP_HWID1_enum"
  UnitConverter_9/1 -> bus_creator/21  "VINP_CrashSignalGPIO_flg"
  UnitConverter_11/1 -> bus_creator/24  "VINP_HWID3_enum"
  UnitConverter_24/1 -> bus_creator/16  "VINP_CentralDoorLockSW_flg"
  UnitConverter_1/1 -> bus_creator/1  "VINP_AccelPedal1VolShortHigh_enum"
  UnitConverter_5/1 -> bus_creator/5  "VINP_AccelPedal2VolShortHigh_enum"
  UnitConverter_26/1 -> bus_creator/18  "VINP_BrakeLampSW_flg"
  UnitConverter_27/1 -> bus_creator/19  "VINP_TrunkHanSW_flg"
  UnitConverter_17/1 -> bus_creator/9  "VINP_BrakeSWGPIO_flg"
  [VINP_TailgateSW_flg] -> UnitConverter_19/1
  UnitConverter_19/1 -> bus_creator/11  "VINP_TailgateSW_flg"
  UnitConverter_21/1 -> bus_creator/13  "VINP_PsDoorSW_flg"
  UnitConverter_22/1 -> bus_creator/14  "VINP_RRDoorSW_flg"
  [VINP_BrakeSWGPIO_flg] -> UnitConverter_17/1
  [VINP_AccelPedal1VolShortLow_enum] -> UnitConverter_2/1
  [VINP_AccelPedal2Vol_V] -> UnitConverter_7/1
  [VINP_CrashSignalGPIO_flg] -> UnitConverter_9/1
  [VINP_DrDoorSW_flg] -> UnitConverter_20/1
  [VINP_PsDoorSW_flg] -> UnitConverter_21/1
  UnitConverter_3/1 -> bus_creator/3  "VINP_AccelPedal1Vol_V"
  bus_creator/1 -> INP_GPIO_outputs/1
  [VINP_AccelPedal2VolShortLow_enum] -> UnitConverter_6/1
  [VINP_AccelPedal2VolShortHigh_enum] -> UnitConverter_5/1
  [VINP_RRDoorSW_flg] -> UnitConverter_22/1
  [VINP_AccelPedal1VolShortHigh_enum] -> UnitConverter_1/1
  [VINP_CentralDoorLockSW_flg] -> UnitConverter_24/1
  UnitConverter_2/1 -> bus_creator/2  "VINP_AccelPedal1VolShortLow_enum"
  UnitConverter_7/1 -> bus_creator/7  "VINP_AccelPedal2Vol_V"
  [VINP_AccelPedal1Vol_V] -> UnitConverter_3/1
  [VINP_RLDoorSW_flg] -> UnitConverter_23/1
  [VINP_AccelPedal1VolValid_flg] -> UnitConverter_4/1
  [VINP_HWID1_enum] -> UnitConverter_69/1
  [VINP_HoodSW_flg] -> UnitConverter_18/1
  [VINP_TrunkHanSW_flg] -> UnitConverter_27/1
  UnitConverter_18/1 -> bus_creator/10  "VINP_HoodSW_flg"
  [VINP_BrakeLampSW_flg] -> UnitConverter_26/1
  UnitConverter_8/1 -> bus_creator/8  "VINP_AccelPedal2VolValid_flg"
  UnitConverter_4/1 -> bus_creator/4  "VINP_AccelPedal1VolValid_flg"
  UnitConverter_6/1 -> bus_creator/6  "VINP_AccelPedal2VolShortLow_enum"
  [VINP_HazardSW_flg] -> UnitConverter_25/1
  UnitConverter_20/1 -> bus_creator/12  "VINP_DrDoorSW_flg"
  UnitConverter_25/1 -> bus_creator/17  "VINP_HazardSW_flg"

== system inp/INP/IMU ==
  BHAL_IMU_outputs : Inport
  Bus Creator : BusCreator  Inputs=12
  Bus Selector : BusSelector  OutputSignals=VHAL_MemOffsetGyroX_raw16,VHAL_MemOffsetGyroY_raw16,VHAL_MemOffsetGyroZ_raw16,VHAL_MemOffsetAccX_raw16,VHAL_MemOffsetAccY_raw16,VHAL_MemOffsetAccZ_raw16,VHAL_SensingGyroX_raw16,VHAL_SensingGyroY_raw16,VHAL_SensingGyroZ_raw16,VHAL_SensingAccX_raw16,VHAL_SensingAccY_raw16,VHAL_SensingAccZ_raw16
  Subsystem1 : Subsystem
  Subsystem10 : Subsystem
  Subsystem11 : Subsystem
  Subsystem15 : Subsystem
  Subsystem2 : Subsystem
  Subsystem3 : Subsystem
  Subsystem4 : Subsystem
  Subsystem5 : Subsystem
  Subsystem6 : Subsystem
  Subsystem7 : Subsystem
  Subsystem8 : Subsystem
  Subsystem9 : Subsystem
  BINP_IMU_outputs : Outport
  wires:
  BHAL_IMU_outputs/1 -> Bus Selector/1
  Bus Selector/1 -> Subsystem15/1(In1)  "<VHAL_MemOffsetGyroX_raw16>"
  Bus Selector/2 -> Subsystem1/1(In1)  "<VHAL_MemOffsetGyroY_raw16>"
  Bus Selector/3 -> Subsystem3/1(In1)  "<VHAL_MemOffsetGyroZ_raw16>"
  Bus Selector/4 -> Subsystem2/1(In1)  "<VHAL_MemOffsetAccX_raw16>"
  Bus Selector/5 -> Subsystem5/1(In1)  "<VHAL_MemOffsetAccY_raw16>"
  Bus Selector/6 -> Subsystem4/1(In1)  "<VHAL_MemOffsetAccZ_raw16>"
  Bus Selector/7 -> Subsystem7/1(In1)  "<VHAL_SensingGyroX_raw16>"
  Bus Selector/8 -> Subsystem6/1(In1)  "<VHAL_SensingGyroY_raw16>"
  Bus Selector/11 -> Subsystem11/1(In1)  "<VHAL_SensingAccY_raw16>"
  Bus Selector/10 -> Subsystem8/1(In1)  "<VHAL_SensingAccX_raw16>"
  Bus Selector/9 -> Subsystem9/1(In1)  "<VHAL_SensingGyroZ_raw16>"
  Bus Selector/12 -> Subsystem10/1(In1)  "<VHAL_SensingAccZ_raw16>"
  Subsystem15/1(Out1) -> Bus Creator/1  "VINP_MemOffsetGyroX_raw16"
  Subsystem1/1(Out1) -> Bus Creator/2  "VINP_MemOffsetGyroY_raw16"
  Subsystem3/1(Out1) -> Bus Creator/3  "VINP_MemOffsetGyroZ_raw16"
  Subsystem2/1(Out1) -> Bus Creator/4  "VINP_MemOffsetAccX_raw16"
  Subsystem5/1(Out1) -> Bus Creator/5  "VINP_MemOffsetAccY_raw16"
  Subsystem4/1(Out1) -> Bus Creator/6  "VINP_MemOffsetAccZ_raw16"
  Subsystem7/1(Out1) -> Bus Creator/7  "VINP_SensingGyroX_raw16"
  Subsystem6/1(Out1) -> Bus Creator/8  "VINP_SensingGyroY_raw16"
  Subsystem9/1(Out1) -> Bus Creator/9  "VINP_SensingGyroZ_raw16"
  Subsystem8/1(Out1) -> Bus Creator/10  "VINP_SensingAccX_raw16"
  Subsystem11/1(Out1) -> Bus Creator/11  "VINP_SensingAccY_raw16"
  Subsystem10/1(Out1) -> Bus Creator/12  "VINP_SensingAccZ_raw16"
  Bus Creator/1 -> BINP_IMU_outputs/1
